simulink model "Design_DC_SERVOMOTOR"  (R2017b)
settings: Solver=VariableStepAuto  StartTime=0.0  StopTime=10.0  RelTol=1e-3
settings Model: Creator=JAY  LastModifiedBy=JAY

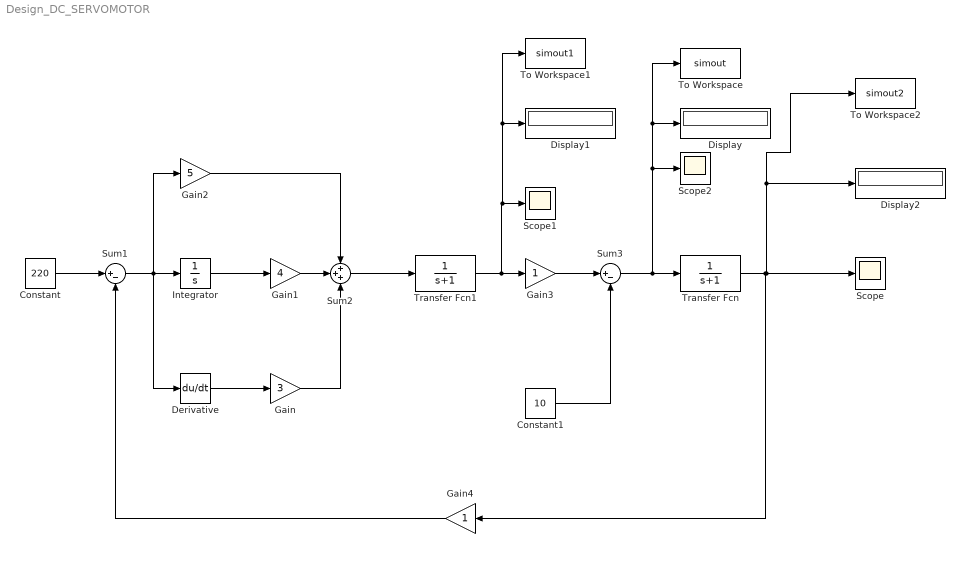
== system Design_DC_SERVOMOTOR ==
  Constant : Constant  Value=220
  Constant1 : Constant  Value=10
  Derivative : Derivative
  Display : Display
  Display1 : Display
  Display2 : Display
  Gain : Gain  Gain=3
  Gain1 : Gain  Gain=4
  Gain2 : Gain  Gain=5
  Gain3 : Gain
  Gain4 : Gain
  Integrator : Integrator
  Scope : Scope
  Scope1 : Scope
  Scope2 : Scope
  Sum1 : Sum  Inputs=|+-
  Sum2 : Sum  Inputs=+++
  Sum3 : Sum  Inputs=|+-
  To Workspace : ToWorkspace  VariableName=simout  SaveFormat=Timeseries  SampleTime=-1
  To Workspace1 : ToWorkspace  VariableName=simout1  SaveFormat=Timeseries  SampleTime=-1
  To Workspace2 : ToWorkspace  VariableName=simout2  SaveFormat=Timeseries  SampleTime=-1
  Transfer Fcn : TransferFcn  Denominator=[1 1]
  Transfer Fcn1 : TransferFcn  Denominator=[1 1]
  wires:
  Constant/1 -> Sum1/1
  Integrator/1 -> Gain1/1
  Sum1/1 -> Derivative/1, Gain2/1, Integrator/1
  Derivative/1 -> Gain/1
  Gain2/1 -> Sum2/1
  Gain1/1 -> Sum2/2
  Sum2/1 -> Transfer Fcn1/1
  Gain/1 -> Sum2/3
  Transfer Fcn1/1 -> Display1/1, To Workspace1/1, Scope1/1, Gain3/1
  Gain3/1 -> Sum3/1
  Gain4/1 -> Sum1/2
  Constant1/1 -> Sum3/2
  Sum3/1 -> Scope2/1, Display/1, To Workspace/1, Transfer Fcn/1
  Transfer Fcn/1 -> To Workspace2/1, Display2/1, Scope/1, Gain4/1
